simulink model "model"  (R2019a)
settings: Solver=FixedStepDiscrete  StartTime=0.0  StopTime=8  FixedStep=1/30  RelTol=1e-3  EnableMultiTasking=on
values from neighbouring files (symbols this model uses):
  A0 = 914.02    [parameter.mat]
  A1 = 12.9    [parameter.mat]
  A2 = 2028.24    [parameter.mat]
  b = 1.14    [parameter.mat]
  bpitch = 4000    [parameter.mat]
  broll = 4000    [parameter.mat]
  c = 1.14    [parameter.mat]
  C1 = 1    [parameter.mat]
  C2 = 0.34    [parameter.mat]
  C3 = 0.57    [parameter.mat]
  C4 = 0.32    [parameter.mat]
  CF = 18.7    [parameter.mat]
  f = 1.215    [parameter.mat]
  Fzt = 810    [parameter.mat]
  hs = 0.55    [parameter.mat]
  ip = 50    [parameter.mat]
  ir = 425    [parameter.mat]
  iw = 1.1    [parameter.mat]
  iz = 3136    [parameter.mat]
  Ka = 0.05    [parameter.mat]
  kpitch = 170000    [parameter.mat]
  kroll = 90000    [parameter.mat]
  m = 750    [parameter.mat]
  miudot = 0.85    [parameter.mat]
  ms = 650    [parameter.mat]
  r = 1.205    [parameter.mat]
  rw = 0.237    [parameter.mat]
  Tp = 24    [parameter.mat]
  Tw = 6    [parameter.mat]
  w = 2.28    [parameter.mat]
undefined symbols (not defined in the file or in its folder): DiscIntNeverNeededParam, Rec, SDTV, sigbuilder_block
libraries: dspmtrx3 x3, visionconversions x2, visiontextngfix x2, visiontransforms x2, fuzblock x1, dspvision x1, visionfilter x1, visionsinks x1, visionstatistics x1
(part 3 of 3)

== system model/Model-based Vehicle Model Subsystem/Tire Model/Subsystem3/Subsystem2 ==
  Fz : Inport
  apdot : Inport  Port=2
  Constant : Constant  Value=CF
  Constant1 : Constant  Value=2
  Divide : Product  Inputs=*/
  Math Function : Math  Operator=square  SaturateOnIntegerOverflow=on
  Product : Product  RndMeth=Zero
  Product1 : Product  RndMeth=Zero
  Kc : Outport
  wires:
  Constant/1 -> Product/1
  Fz/1 -> Product/2
  apdot/1 -> Math Function/1
  Constant1/1 -> Divide/1
  Math Function/1 -> Divide/2
  Product/1 -> Product1/1
  Divide/1 -> Product1/2
  Product1/1 -> Kc/1

== system model/Model-based Vehicle Model Subsystem/Tire Model/Subsystem3/Subsystem3 ==
  Fz : Inport
  apdot : Inport  Port=2
  Add : Sum
  Constant : Constant  Value=A0
  Constant1 : Constant  Value=A1
  Constant2 : Constant  Value=A1
  Constant3 : Constant  Value=A2
  Constant4 : Constant  Value=2
  Divide : Product  Inputs=*/
  Divide1 : Product  Inputs=*/
  Math Function : Math  Operator=square  SaturateOnIntegerOverflow=on
  Math Function1 : Math  Operator=square  SaturateOnIntegerOverflow=on
  Product : Product  RndMeth=Zero
  Product1 : Product  RndMeth=Zero
  Product2 : Product  RndMeth=Zero
  Terminator : Terminator
  Ks : Outport
  wires:
  Constant/1 -> Add/1
  Product/1 -> Add/2
  Constant1/1 -> Product/1
  Fz/1 -> Product/2, Math Function/1
  Constant2/1 -> Divide/1
  Constant3/1 -> Divide/2
  Divide/1 -> Product1/1
  Math Function/1 -> Product1/2
  Divide1/1 -> Product2/2
  Add/1 -> Product2/1
  Constant4/1 -> Divide1/1
  apdot/1 -> Math Function1/1
  Math Function1/1 -> Divide1/2
  Product2/1 -> Ks/1
  Product1/1 -> Terminator/1

== system model/Model-based Vehicle Model Subsystem/Tire Model/Subsystem3/Subsystem4 ==
  ap : Inport
  Fz : Inport  Port=2
  Ks : Inport  Port=3
  Kc : Inport  Port=4
  s : Inport  Port=5
  Alpha : Inport  Port=6
  Add : Sum
  Constant : Constant
  Constant1 : Constant  Value=pi
  Constant2 : Constant  Value=8
  Constant3 : Constant  Value=miudot
  Divide : Product  Inputs=*/
  Divide1 : Product  Inputs=*/
  Math Function{,1,3..5} (5 alike) : Math  Operator=square  SaturateOnIntegerOverflow=on
  Math Function2 : Math  Operator=sqrt  SaturateOnIntegerOverflow=on
  Product{,1..2,4} (4 alike) : Product  RndMeth=Zero
  Product3 : Product  Inputs=3  RndMeth=Zero
  Subtract : Sum  Inputs=-+
  Trigonometric Function : Trigonometry  Operator=tan
  gama : Outport
  wires:
  Constant/1 -> Subtract/2
  s/1 -> Subtract/1, Divide/1
  Subtract/1 -> Divide/2
  Divide/1 -> Math Function/1
  Kc/1 -> Math Function1/1
  Math Function1/1 -> Product/1
  Math Function/1 -> Product/2
  Product/1 -> Add/2
  Add/1 -> Math Function2/1
  Alpha/1 -> Trigonometric Function/1
  Trigonometric Function/1 -> Math Function3/1
  Math Function3/1 -> Product1/1
  Ks/1 -> Math Function4/1
  Math Function4/1 -> Product1/2
  Product1/1 -> Add/1
  Constant1/1 -> Product2/1
  ap/1 -> Math Function5/1
  Math Function5/1 -> Product2/2
  Product2/1 -> Divide1/1
  Fz/1 -> Product3/1
  Product3/1 -> Divide1/2
  Constant2/1 -> Product3/2
  Constant3/1 -> Product3/3
  Product4/1 -> gama/1
  Divide1/1 -> Product4/1
  Math Function2/1 -> Product4/2

== system model/Model-based Vehicle Model Subsystem/Tire Model/Subsystem3/Subsystem5 ==
  gama : Inport
  Add : Sum  Inputs=+++
  Add1 : Sum  Inputs=++++
  Constant : Constant  Value=C1
  Constant1 : Constant  Value=C2
  Constant2 : Constant  Value=C3
  Constant3 : Constant  Value=C4
  Constant4 : Constant  Value=4
  Constant5 : Constant  Value=pi
  Constant6 : Constant
  Divide : Product  Inputs=*/
  Divide1 : Product  Inputs=*/
  Math Function : Math  Operator=square  SaturateOnIntegerOverflow=on
  Product{,1..5} (6 alike) : Product  RndMeth=Zero
  f(gama) : Outport
  wires:
  gama/1 -> Math Function/1, Product/2, Product3/1, Product5/1
  Math Function/1 -> Product/1, Product2/2, Product4/1
  Product/1 -> Product1/1
  Constant/1 -> Product1/2
  Product1/1 -> Add/1, Add1/1
  Constant1/1 -> Product2/1
  Product2/1 -> Add/2
  Constant4/1 -> Divide/1
  Constant5/1 -> Divide/2
  Divide/1 -> Product3/2
  Product3/1 -> Add/3
  Constant2/1 -> Product4/2
  Product4/1 -> Add1/2
  Product5/1 -> Add1/3
  Constant3/1 -> Product5/2
  Constant6/1 -> Add1/4
  Add/1 -> Divide1/1
  Add1/1 -> Divide1/2
  Divide1/1 -> f(gama)/1

== system model/Model-based Vehicle Model Subsystem/Tire Model/Subsystem3/Subsystem6 ==
  Kc : Inport
  Ks : Inport  Port=2
  s : Inport  Port=3
  Alpha : Inport  Port=4
  Add : Sum
  Add1 : Sum
  Math Function : Math  Operator=square  SaturateOnIntegerOverflow=on
  Math Function1 : Math  Operator=square  SaturateOnIntegerOverflow=on
  Math Function2 : Math  Operator=sqrt  SaturateOnIntegerOverflow=on
  Math Function3 : Math  Operator=square  SaturateOnIntegerOverflow=on
  Product : Product  RndMeth=Zero
  Product1 : Product  RndMeth=Zero
  Subtract : Sum  Inputs=+-
  Trigonometric Function : Trigonometry  Operator=cos
  Trigonometric Function1 : Trigonometry
  K'c : Outport
  wires:
  s/1 -> Math Function/1
  Alpha/1 -> Trigonometric Function/1, Trigonometric Function1/1
  Trigonometric Function/1 -> Math Function1/1
  Math Function1/1 -> Product/2
  Math Function/1 -> Product/1
  Product/1 -> Add/2
  Add/1 -> Math Function2/1
  Trigonometric Function1/1 -> Math Function3/1
  Math Function3/1 -> Add/1
  Math Function2/1 -> Product1/2
  Ks/1 -> Subtract/1
  Kc/1 -> Subtract/2, Add1/1
  Subtract/1 -> Product1/1
  Product1/1 -> Add1/2
  Add1/1 -> K'c/1

== system model/Model-based Vehicle Model Subsystem/Tire Model/Subsystem3/Subsystem7 ==
  K'c : Inport
  Fz : Inport  Port=2
  s : Inport  Port=3
  Ks : Inport  Port=4
  f(gama) : Inport  Port=5
  Alpha : Inport  Port=6
  Add : Sum
  Divide : Product  Inputs=*/
  Gain : Gain  Gain=0.85
  Math Function{,1..3} (4 alike) : Math  Operator=square  SaturateOnIntegerOverflow=on
  Math Function4 : Math  Operator=sqrt  SaturateOnIntegerOverflow=on
  Product : Product  RndMeth=Zero
  Product1 : Product  RndMeth=Zero
  Product2 : Product  Inputs=4  RndMeth=Zero
  Subsystem : Subsystem
  Trigonometric Function : Trigonometry  Operator=tan
  Fx : Outport
  out1 : Outport  Port=2
  out2 : Outport  Port=3
  wires:
  Ks/1 -> Math Function/1
  Math Function/1 -> Product/1
  Alpha/1 -> Trigonometric Function/1
  Trigonometric Function/1 -> Math Function1/1
  Math Function1/1 -> Product/2
  Product/1 -> Add/1
  K'c/1 -> Math Function2/1, Product2/4
  s/1 -> Math Function3/1, Product2/3
  Math Function2/1 -> Product1/1
  Math Function3/1 -> Product1/2
  Product1/1 -> Add/2
  Add/1 -> Math Function4/1
  Product2/1 -> Divide/1
  Fz/1 -> Gain/1
  f(gama)/1 -> Product2/2
  Divide/1 -> Fx/1
  Math Function4/1 -> Subsystem/1(In1)
  Gain/1 -> Product2/1, out2/1
  Subsystem/1(Out1) -> Divide/2, out1/1

== system model/Model-based Vehicle Model Subsystem/Tire Model/Subsystem3/Subsystem8 ==
  in1 : Inport
  in2 : Inport  Port=2
  Ks : Inport  Port=3
  f(gama) : Inport  Port=4
  Alpha : Inport  Port=5
  Divide : Product  Inputs=*/
  Gain3 : Gain  Gain=-1
  Product2 : Product  Inputs=4  RndMeth=Zero
  Trigonometric Function : Trigonometry  Operator=tan
  Fy : Outport
  wires:
  Ks/1 -> Product2/4
  Alpha/1 -> Trigonometric Function/1
  Trigonometric Function/1 -> Product2/3
  Product2/1 -> Divide/1
  f(gama)/1 -> Product2/2
  Divide/1 -> Gain3/1
  in2/1 -> Product2/1
  in1/1 -> Divide/2
  Gain3/1 -> Fy/1

== system model/Model-based Vehicle Model Subsystem/Tire Model/Subsystem/Subsystem7/Subsystem ==
  In1 : Inport
  Constant : Constant  Value=0.01
  Constant1 : Constant  Value=-0.01
  If : If  IfExpression=0<u1 & u1<= 0.01  ElseIfExpressions=-0.01<u1 & u1<=0
  If Action Subsystem : Subsystem  TreatAsAtomicUnit=on
  If Action Subsystem1 : Subsystem  TreatAsAtomicUnit=on
  If Action Subsystem2 : Subsystem  TreatAsAtomicUnit=on
  Merge : Merge  Inputs=3
  Out1 : Outport
  wires:
  If/1 -> If Action Subsystem/Action
  Constant/1 -> If Action Subsystem/1(In1)
  If Action Subsystem/1(Out1) -> Merge/1
  If/2 -> If Action Subsystem1/Action
  Constant1/1 -> If Action Subsystem1/1(In1)
  If/3 -> If Action Subsystem2/Action
  In1/1 -> If Action Subsystem2/1(In1), If/1
  If Action Subsystem1/1(Out1) -> Merge/2
  If Action Subsystem2/1(Out1) -> Merge/3
  Merge/1 -> Out1/1

== system model/Model-based Vehicle Model Subsystem/Tire Model/Subsystem1/Subsystem7/Subsystem ==
  In1 : Inport
  Constant : Constant  Value=0.01
  Constant1 : Constant  Value=-0.01
  If : If  IfExpression=0<u1 & u1<= 0.01  ElseIfExpressions=-0.01<u1 & u1<=0
  If Action Subsystem : Subsystem  TreatAsAtomicUnit=on
  If Action Subsystem1 : Subsystem  TreatAsAtomicUnit=on
  If Action Subsystem2 : Subsystem  TreatAsAtomicUnit=on
  Merge : Merge  Inputs=3
  Out1 : Outport
  wires:
  If/1 -> If Action Subsystem/Action
  Constant/1 -> If Action Subsystem/1(In1)
  If Action Subsystem/1(Out1) -> Merge/1
  If/2 -> If Action Subsystem1/Action
  Constant1/1 -> If Action Subsystem1/1(In1)
  If/3 -> If Action Subsystem2/Action
  In1/1 -> If Action Subsystem2/1(In1), If/1
  If Action Subsystem1/1(Out1) -> Merge/2
  If Action Subsystem2/1(Out1) -> Merge/3
  Merge/1 -> Out1/1

== system model/Model-based Vehicle Model Subsystem/Tire Model/Subsystem2/Subsystem7/Subsystem ==
  In1 : Inport
  Constant : Constant  Value=0.01
  Constant1 : Constant  Value=-0.01
  If : If  IfExpression=0<u1 & u1<= 0.01  ElseIfExpressions=-0.01<u1 & u1<=0
  If Action Subsystem : Subsystem  TreatAsAtomicUnit=on
  If Action Subsystem1 : Subsystem  TreatAsAtomicUnit=on
  If Action Subsystem2 : Subsystem  TreatAsAtomicUnit=on
  Merge : Merge  Inputs=3
  Out1 : Outport
  wires:
  If/1 -> If Action Subsystem/Action
  Constant/1 -> If Action Subsystem/1(In1)
  If Action Subsystem/1(Out1) -> Merge/1
  If/2 -> If Action Subsystem1/Action
  Constant1/1 -> If Action Subsystem1/1(In1)
  If/3 -> If Action Subsystem2/Action
  In1/1 -> If Action Subsystem2/1(In1), If/1
  If Action Subsystem1/1(Out1) -> Merge/2
  If Action Subsystem2/1(Out1) -> Merge/3
  Merge/1 -> Out1/1

== system model/Model-based Vehicle Model Subsystem/Tire Model/Subsystem3/Subsystem7/Subsystem ==
  In1 : Inport
  Constant : Constant  Value=0.01
  Constant1 : Constant  Value=-0.01
  If : If  IfExpression=0<u1 & u1<= 0.01  ElseIfExpressions=-0.01<u1 & u1<=0
  If Action Subsystem : Subsystem  TreatAsAtomicUnit=on
  If Action Subsystem1 : Subsystem  TreatAsAtomicUnit=on
  If Action Subsystem2 : Subsystem  TreatAsAtomicUnit=on
  Merge : Merge  Inputs=3
  Out1 : Outport
  wires:
  If/1 -> If Action Subsystem/Action
  Constant/1 -> If Action Subsystem/1(In1)
  If Action Subsystem/1(Out1) -> Merge/1
  If/2 -> If Action Subsystem1/Action
  Constant1/1 -> If Action Subsystem1/1(In1)
  If/3 -> If Action Subsystem2/Action
  In1/1 -> If Action Subsystem2/1(In1), If/1
  If Action Subsystem1/1(Out1) -> Merge/2
  If Action Subsystem2/1(Out1) -> Merge/3
  Merge/1 -> Out1/1

== system model/Model-based Vehicle Model Subsystem/Tire Model/Subsystem/Subsystem7/Subsystem/If Action Subsystem ==
  In1 : Inport
  Action Port : ActionPort  PropagateVarSize=During execution  ActionPortLabel=if { }
  Out1 : Outport
  wires:
  In1/1 -> Out1/1

== system model/Model-based Vehicle Model Subsystem/Tire Model/Subsystem/Subsystem7/Subsystem/If Action Subsystem1 ==
  In1 : Inport
  Action Port : ActionPort  PropagateVarSize=During execution  ActionPortLabel=elseif { }
  Out1 : Outport
  wires:
  In1/1 -> Out1/1

== system model/Model-based Vehicle Model Subsystem/Tire Model/Subsystem/Subsystem7/Subsystem/If Action Subsystem2 ==
  In1 : Inport
  Action Port : ActionPort  PropagateVarSize=During execution  ActionPortLabel=else { }
  Out1 : Outport
  wires:
  In1/1 -> Out1/1

== system model/Model-based Vehicle Model Subsystem/Tire Model/Subsystem1/Subsystem7/Subsystem/If Action Subsystem ==
  In1 : Inport
  Action Port : ActionPort  PropagateVarSize=During execution  ActionPortLabel=if { }
  Out1 : Outport
  wires:
  In1/1 -> Out1/1

== system model/Model-based Vehicle Model Subsystem/Tire Model/Subsystem1/Subsystem7/Subsystem/If Action Subsystem1 ==
  In1 : Inport
  Action Port : ActionPort  PropagateVarSize=During execution  ActionPortLabel=elseif { }
  Out1 : Outport
  wires:
  In1/1 -> Out1/1

== system model/Model-based Vehicle Model Subsystem/Tire Model/Subsystem1/Subsystem7/Subsystem/If Action Subsystem2 ==
  In1 : Inport
  Action Port : ActionPort  PropagateVarSize=During execution  ActionPortLabel=else { }
  Out1 : Outport
  wires:
  In1/1 -> Out1/1

== system model/Model-based Vehicle Model Subsystem/Tire Model/Subsystem2/Subsystem7/Subsystem/If Action Subsystem ==
  In1 : Inport
  Action Port : ActionPort  PropagateVarSize=During execution  ActionPortLabel=if { }
  Out1 : Outport
  wires:
  In1/1 -> Out1/1

== system model/Model-based Vehicle Model Subsystem/Tire Model/Subsystem2/Subsystem7/Subsystem/If Action Subsystem1 ==
  In1 : Inport
  Action Port : ActionPort  PropagateVarSize=During execution  ActionPortLabel=elseif { }
  Out1 : Outport
  wires:
  In1/1 -> Out1/1

== system model/Model-based Vehicle Model Subsystem/Tire Model/Subsystem2/Subsystem7/Subsystem/If Action Subsystem2 ==
  In1 : Inport
  Action Port : ActionPort  PropagateVarSize=During execution  ActionPortLabel=else { }
  Out1 : Outport
  wires:
  In1/1 -> Out1/1

== system model/Model-based Vehicle Model Subsystem/Tire Model/Subsystem3/Subsystem7/Subsystem/If Action Subsystem ==
  In1 : Inport
  Action Port : ActionPort  PropagateVarSize=During execution  ActionPortLabel=if { }
  Out1 : Outport
  wires:
  In1/1 -> Out1/1

== system model/Model-based Vehicle Model Subsystem/Tire Model/Subsystem3/Subsystem7/Subsystem/If Action Subsystem1 ==
  In1 : Inport
  Action Port : ActionPort  PropagateVarSize=During execution  ActionPortLabel=elseif { }
  Out1 : Outport
  wires:
  In1/1 -> Out1/1

== system model/Model-based Vehicle Model Subsystem/Tire Model/Subsystem3/Subsystem7/Subsystem/If Action Subsystem2 ==
  In1 : Inport
  Action Port : ActionPort  PropagateVarSize=During execution  ActionPortLabel=else { }
  Out1 : Outport
  wires:
  In1/1 -> Out1/1
